simulink model "VXRv1 (1)"  (R2020b)
settings: Solver=VariableStepAuto  StartTime=0.0  StopTime=0.5  RelTol=1e-3
libraries: fl_lib x62, ee_lib x36, nesl_utility x19, powerlib_meascontrol x6
settings Model: Creator=Admin  LastModifiedBy=olivermizzaro

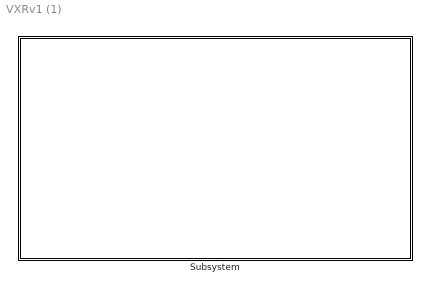
== system VXRv1 (1) ==
  Subsystem : Subsystem

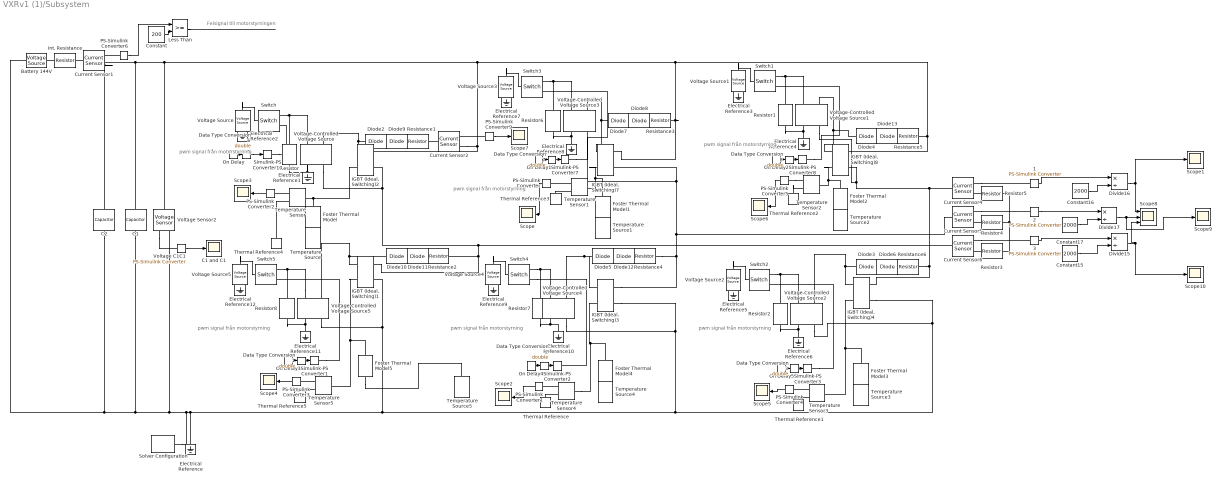
== system VXRv1 (1)/Subsystem ==
  note: pwm signal från motorstyrning
  note: Felsignal till motorstyrningen
  note: pwm signal från motorstyrning
  note: pwm signal från motorstyrning
  note: pwm signal från motorstyrning
  note: pwm signal från motorstyrning
  note: pwm signal från motorstyrning
   Resistance{1..6} (6 alike) : fl_lib/Electrical/Electrical Elements/Resistor  R=30 Ohm  i_specify=off  i_priority=None  i=0 A  i_nominal_specify=off  i_nominal_unit=A  i_nominal_value=1  v_specify=off  v_priority=None  v=0 V  v_nominal_specify=off  v_nominal_unit=V  v_nominal_value=1
  1 : nesl_utility/PS-Simulink Converter  PhysicalDomain=network_engine_domain  SubClassName=ps_output  LeftPortType=input  RightPortType=output  PseudoPeriodic=off  Frequencies=[]  Unit=inherit  AffineConversion=off
  2 : nesl_utility/PS-Simulink Converter  PhysicalDomain=network_engine_domain  SubClassName=ps_output  LeftPortType=input  RightPortType=output  PseudoPeriodic=off  Frequencies=[]  Unit=inherit  AffineConversion=off
  3 : nesl_utility/PS-Simulink Converter  PhysicalDomain=network_engine_domain  SubClassName=ps_output  LeftPortType=input  RightPortType=output  PseudoPeriodic=off  Frequencies=[]  Unit=inherit  AffineConversion=off
  Battery 144V : ee_lib/Sources/Voltage Source  dc_voltage=144 V  ac_voltage=0 V  ac_shift=0 rad  ac_frequency=60 Hz  noise_mode=0  PSD=0 V^2/Hz  repeatability=1  auto_seed=785646024  user_seed=0  sample_time=1e-3 s  i_specify=off  i_priority=None  i=0 A  i_nominal_specify=off  i_nominal_unit=A  i_nominal_value=1  v_specify=off  v_priority=None  v=0 V  v_nominal_specify=off  v_nominal_unit=V  v_nominal_value=1
  C1 : ee_lib/Passive/Capacitor  cap_option=0  c=10000e-6 F  Cvec=[1e-05, 1e-06] F  Vvec=[0, 10] V  CV_table_symmetry=1  f_vec=[1, 10] kHz  DFext_vec=[.8, 1.2]  C_tol=5  enable_C_tol=0  tol_distribution=1  nSigma=4  r=1 Ohm  g=0 1/Ohm  averaging_period=0 s  enable_operating_limits=0  operating_limit_action=2  max_working_voltage_range=[-25, 25] V  power_rating=1 W  enable_faults=0  fault_action=1  Cscale_faulted=100  R_faulted=1e-3 Ohm  G_faulted=0 1/Ohm  tau_fault=1e-3 s  enable_temporal_fault=0  t_fault=1 s  enable_behavioral_fault=0  max_permissible_voltage_range=[-100, 100] V  t_fail_on_voltage=1 s  i_specify=off  i_priority=None  i=0 A  i_nominal_specify=off  i_nominal_unit=A  i_nominal_value=1  v_specify=off  v_priority=None  v=0 V  v_nominal_specify=off  v_nominal_unit=V  v_nominal_value=1  vc_specify=on  vc_priority=High  vc=144 V  vc_nominal_specify=off  vc_nominal_unit=V  vc_nominal_value=1
  C1 and C1 : Scope
  C2 : ee_lib/Passive/Capacitor  cap_option=0  c=127e-9 F  Cvec=[1e-05, 1e-06] F  Vvec=[0, 10] V  CV_table_symmetry=1  f_vec=[1, 10] kHz  DFext_vec=[.8, 1.2]  C_tol=5  enable_C_tol=0  tol_distribution=1  nSigma=4  r=1 Ohm  g=0 1/Ohm  averaging_period=0 s  enable_operating_limits=0  operating_limit_action=2  max_working_voltage_range=[-25, 25] V  power_rating=1 W  enable_faults=0  fault_action=1  Cscale_faulted=100  R_faulted=1e-3 Ohm  G_faulted=0 1/Ohm  tau_fault=1e-3 s  enable_temporal_fault=0  t_fault=1 s  enable_behavioral_fault=0  max_permissible_voltage_range=[-100, 100] V  t_fail_on_voltage=1 s  i_specify=off  i_priority=None  i=0 A  i_nominal_specify=off  i_nominal_unit=A  i_nominal_value=1  v_specify=off  v_priority=None  v=0 V  v_nominal_specify=off  v_nominal_unit=V  v_nominal_value=1  vc_specify=off  vc_priority=High  vc=0 V  vc_nominal_specify=off  vc_nominal_unit=V  vc_nominal_value=1
  Constant : Constant  Value=200
  Constant15 : Constant  Value=2000
  Constant16 : Constant  Value=2000
  Constant17 : Constant  Value=2000
  Current Sensor{1..2,4..6} (5 alike) : fl_lib/Electrical/Electrical Sensors/Current Sensor
  Data Type Conversion{1..3,6..8} (6 alike) : DataTypeConversion  OutDataTypeStr=double
  Diode{2..5,7,10} (6 alike) : ee_lib/Semiconductors & Converters/Diode  ModelType=ee.enum.diode.modelType.pwl  IfMat=[.07, .12, .19, 1.75, 4.24, 7.32, 11.2; .16, .3, .72, 2.14, 4.02, 6.35, 9.12] A  TjVec=[25, 125] degC  VfVec=[.5, .7, .9, 1.3, 1.7, 2.1, 2.5] V  Vf=3 V  Ron=5 Ohm  Goff=1e-8 S  prmExp=ee.enum.diode.expParam.useTwo  I12=[.0137, .545] A  V12=[.6, .7] V  IS=1e-12 A  ec=1  I1=0.0137 A  V1=0.6 V  RS=0 Ohm  Tmeas=25 degC  N_series=1  N_parallel=1  Rz=1.5 Ohm  BV=150 V  C_param=ee.enum.diode.capParam.fixed  CJ=5 pF  CJ0=5 pF  VJ=1 V  Mgrad=0.5  Vvec=[.1, 10, 100] V  Cvec=[3.5, 1, .4] pF  FC=0.5  Q_param=ee.enum.diode.recoveryParam.off  iRM=-7.15 A  iF=4 A  didt=-750 A/us  trr_factor=3  trr=115 ns  Qrr=1500 s*uA  TT=50 ns  tau=100 ns  T_param=ee.enum.diode.temperatureParam.off  IS_T2=1.25e-7 A  I1_T2=0.245 A  V1_T2=0.5 V  Tmeas2=125 degC  EG_param=ee.enum.diode.egapParam.material_si  EG=1.11 eV  XTI_param=ee.enum.diode.xtiParam.pn  XTI=3  dBVdT=0 V/K  Tdevice=25 degC  i_specify=off  i_priority=None  i=0 A  i_nominal_specify=off  i_nominal_unit=A  i_nominal_value=1  v_specify=off  v_priority=None  v=0 V  v_nominal_specify=off  v_nominal_unit=V  v_nominal_value=1  i_capacitor_specify=off  i_capacitor_priority=None  i_capacitor=0 A  i_capacitor_nominal_specify=off  i_capacitor_nominal_unit=A  i_capacitor_nominal_value=1  v_capacitor_specify=off  v_capacitor_priority=None  v_capacitor=0 V  v_capacitor_nominal_specify=off  v_capacitor_nominal_unit=V  v_capacitor_nominal_value=1  power_dissipated_specify=off  power_dissipated_priority=None  power_dissipated=0 W  power_dissipated_nominal_specify=off  power_dissipated_nominal_unit=W  power_dissipated_nominal_value=1  thermal_network_parameterization=ee.enum.thermalNetworkTopology.cauer  Rth=[0, 10] K/W  Rth_Foster=[4, 6] K/W  thermal_mass_parameterization=ee.enum.thermalNetwork.timeconstant  thermal_mass=[0, 1] J/K  thermal_mass_Foster=[1.5, 3] J/K  thermal_time_constant=[0, 10] s  thermal_time_constant_Foster=[6, 18] s  thermal_mass_initial_temperatures=[25, 25] degC
  Diode{6,8..9,11..13} (6 alike) : ee_lib/Semiconductors & Converters/Diode  ModelType=ee.enum.diode.modelType.pwl  IfMat=[.07, .12, .19, 1.75, 4.24, 7.32, 11.2; .16, .3, .72, 2.14, 4.02, 6.35, 9.12] A  TjVec=[25, 125] degC  VfVec=[.5, .7, .9, 1.3, 1.7, 2.1, 2.5] V  Vf=0.6 V  Ron=0.3 Ohm  Goff=1e-8 S  prmExp=ee.enum.diode.expParam.useTwo  I12=[.0137, .545] A  V12=[.6, .7] V  IS=1e-12 A  ec=1  I1=0.0137 A  V1=0.6 V  RS=0 Ohm  Tmeas=25 degC  N_series=1  N_parallel=1  Rz=0.3 Ohm  BV=inf V  C_param=ee.enum.diode.capParam.fixed  CJ=5 pF  CJ0=5 pF  VJ=1 V  Mgrad=0.5  Vvec=[.1, 10, 100] V  Cvec=[3.5, 1, .4] pF  FC=0.5  Q_param=ee.enum.diode.recoveryParam.off  iRM=-7.15 A  iF=4 A  didt=-750 A/us  trr_factor=3  trr=115 ns  Qrr=1500 s*uA  TT=50 ns  tau=100 ns  T_param=ee.enum.diode.temperatureParam.off  IS_T2=1.25e-7 A  I1_T2=0.245 A  V1_T2=0.5 V  Tmeas2=125 degC  EG_param=ee.enum.diode.egapParam.material_si  EG=1.11 eV  XTI_param=ee.enum.diode.xtiParam.pn  XTI=3  dBVdT=0 V/K  Tdevice=25 degC  i_specify=off  i_priority=None  i=0 A  i_nominal_specify=off  i_nominal_unit=A  i_nominal_value=1  v_specify=off  v_priority=None  v=0 V  v_nominal_specify=off  v_nominal_unit=V  v_nominal_value=1  i_capacitor_specify=off  i_capacitor_priority=None  i_capacitor=0 A  i_capacitor_nominal_specify=off  i_capacitor_nominal_unit=A  i_capacitor_nominal_value=1  v_capacitor_specify=off  v_capacitor_priority=None  v_capacitor=0 V  v_capacitor_nominal_specify=off  v_capacitor_nominal_unit=V  v_capacitor_nominal_value=1  power_dissipated_specify=off  power_dissipated_priority=None  power_dissipated=0 W  power_dissipated_nominal_specify=off  power_dissipated_nominal_unit=W  power_dissipated_nominal_value=1  thermal_network_parameterization=ee.enum.thermalNetworkTopology.cauer  Rth=[0, 10] K/W  Rth_Foster=[4, 6] K/W  thermal_mass_parameterization=ee.enum.thermalNetwork.timeconstant  thermal_mass=[0, 1] J/K  thermal_mass_Foster=[1.5, 3] J/K  thermal_time_constant=[0, 10] s  thermal_time_constant_Foster=[6, 18] s  thermal_mass_initial_temperatures=[25, 25] degC
  Divide15 : Product  Inputs=*/
  Divide16 : Product  Inputs=*/
  Divide17 : Product  Inputs=*/
  Electrical Reference{,1..12} (13 alike) : fl_lib/Electrical/Electrical Elements/Electrical Reference
  Foster Thermal Model{,1..5} (6 alike) : ee_lib/Passive/Thermal/Foster Thermal Model  resistance_data=[ 0.0016 0.0043 0.0013 0.0014 ] K/W  tau_data=[ 0.0068 0.064 0.32 2 ] s
      settings: SourceProductBaseCode=PS  InternalSimscapePortConfiguration="{\"Bottom\":[],\"Left\":[{\"id\":\"A\",\"label\":\"A\",\"type\":\"foundation.thermal.thermal\"}],\"Right\":[{\"id\":\"B\",\"label\":\"B\",\"type\":\"foundation.thermal.thermal\"}],\"Top\":[]}"
  IGBT (Ideal, Switching){1,3..4,8} (4 alike) : ee_lib/Semiconductors & Converters/IGBT (Ideal, Switching)  Vf=1.5 V  Ron=0.001 Ohm  Goff=1e-5 1/Ohm  Vth=0.1 V  diode_param=ee.enum.converters.protectiondiode.none  diode_Vf=0.8 V  diode_Ron=0.001 Ohm  diode_Goff=1e-5 1/Ohm  diode_C=50e-9 F  diode_iRM=-235 A  diode_iF=300 A  diode_idot=-50 A/us  diode_trr_param=ee.enum.converters.diodetrr.trr_factor  diode_trr_factor=3  diode_trr=15 us  diode_Qrr=1500 s*uA  thermal_loss_option=ee.enum.converters.thermalLossOption.constantvalues  Von_data=[0, .1, .6, .8, 1, 1.3, 1.6, 2, 2.4; 0, .1, .7, 1, 1.2, 1.5, 1.9, 2.4, 2.8] V  Eon_data=[0, .0024, .024, .12, .2, .48, 1.04, 2.16, 3.24; 0, .003, .03, .15, .25, .6, 1.3, 2.7, 4.05] * 1e-3 J  Eoff_data=[0, .0007, .0066, .033, .066, .17, .33, .83, 1.5; 0, .001, .01, .05, .1, .25, .5, 1.2, 2.2] * 1e-3 J  Tj=[298.15, 398.15] K  Iout_data=[0, .1, 1, 5, 10, 20, 40, 70, 100] A  Eon_scalar=2.9e-3 J  Eoff_scalar=7.9e-3 J  Voff=300 V  Iout_scalar=600 A  diodeModelType=ee.enum.converters.diodeModelType.pwl  diode_IfMat=[.07, .12, .19, 1.75, 4.24, 7.32, 11.2; .16, .3, .72, 2.14, 4.02, 6.35, 9.12] A  diode_TjVec=[25, 125] degC  diode_VfVec=[.5, .7, .9, 1.3, 1.7, 2.1, 2.5] V  thermal_network_parameterization=ee.enum.thermalNetworkTopology.cauer  Rth=[.42, .06] K/W  Rth_Foster=[.08, .14, .22, .16] K/W  thermal_mass_parameterization=ee.enum.thermalNetwork.timeconstant  thermal_mass=[.01, .5] J/K  thermal_mass_Foster=[.001, .005, .05, .5] J/K  thermal_time_constant=[.001, .2] s  thermal_time_constant_Foster=[7e-05, .0007, .01, .08] s  thermal_mass_initial_temperatures=[25, 25] degC  junction_thermal_mass=0.01 J/K  Tau=1e-4 s  vT_specify=off  vT_priority=None  vT=0 V  vT_nominal_specify=off  vT_nominal_unit=V  vT_nominal_value=1  Qj_specify=off  Qj_priority=None  Qj=0 W  Qj_nominal_specify=off  Qj_nominal_unit=W  Qj_nominal_value=1  junction_temperature_specify=off  junction_temperature_priority=None  junction_temperature=25 degC  junction_temperature_nominal_specify=off  junction_temperature_nominal_unit=degC  junction_temperature_nominal_value=1
      settings: InternalSimscapePortConfiguration="{\"Bottom\":[],\"Left\":[{\"id\":\"G\",\"label\":\"\",\"type\":\"foundation.electrical.electrical\"},{\"id\":\"H\",\"label\":\"\",\"type\":\"foundation.thermal.thermal\"}],\"Right\":[{\"id\":\"C\",\"label\":\"\",\"type\":\"foundation.electrical.electrical\"},{\"id\":\"E\",\"label\":\"\",\"type\":\"foundation.electrical.electrical\"}],\"Top\":[]}"
  "IGBT (Ideal, Switching)2" : ee_lib/Semiconductors & Converters/IGBT (Ideal, Switching)  Vf=1.5 V  Ron=0.001 Ohm  Goff=1e-5 1/Ohm  Vth=7 V  diode_param=ee.enum.converters.protectiondiode.none  diode_Vf=0.8 V  diode_Ron=0.001 Ohm  diode_Goff=1e-5 1/Ohm  diode_C=50e-9 F  diode_iRM=-235 A  diode_iF=300 A  diode_idot=-50 A/us  diode_trr_param=ee.enum.converters.diodetrr.trr_factor  diode_trr_factor=3  diode_trr=15 us  diode_Qrr=1500 s*uA  thermal_loss_option=ee.enum.converters.thermalLossOption.constantvalues  Von_data=[0, .1, .6, .8, 1, 1.3, 1.6, 2, 2.4; 0, .1, .7, 1, 1.2, 1.5, 1.9, 2.4, 2.8] V  Eon_data=[0, .0024, .024, .12, .2, .48, 1.04, 2.16, 3.24; 0, .003, .03, .15, .25, .6, 1.3, 2.7, 4.05] * 1e-3 J  Eoff_data=[0, .0007, .0066, .033, .066, .17, .33, .83, 1.5; 0, .001, .01, .05, .1, .25, .5, 1.2, 2.2] * 1e-3 J  Tj=[298.15, 398.15] K  Iout_data=[0, .1, 1, 5, 10, 20, 40, 70, 100] A  Eon_scalar=2.9e-3 J  Eoff_scalar=7.9e-3 J  Voff=300 V  Iout_scalar=600 A  diodeModelType=ee.enum.converters.diodeModelType.pwl  diode_IfMat=[.07, .12, .19, 1.75, 4.24, 7.32, 11.2; .16, .3, .72, 2.14, 4.02, 6.35, 9.12] A  diode_TjVec=[25, 125] degC  diode_VfVec=[.5, .7, .9, 1.3, 1.7, 2.1, 2.5] V  thermal_network_parameterization=ee.enum.thermalNetworkTopology.cauer  Rth=[.42, .06] K/W  Rth_Foster=[.08, .14, .22, .16] K/W  thermal_mass_parameterization=ee.enum.thermalNetwork.timeconstant  thermal_mass=[.01, .5] J/K  thermal_mass_Foster=[.001, .005, .05, .5] J/K  thermal_time_constant=[.001, .2] s  thermal_time_constant_Foster=[7e-05, .0007, .01, .08] s  thermal_mass_initial_temperatures=[25, 25] degC  junction_thermal_mass=0.01 J/K  Tau=1e-4 s  vT_specify=off  vT_priority=None  vT=0 V  vT_nominal_specify=off  vT_nominal_unit=V  vT_nominal_value=1  Qj_specify=off  Qj_priority=None  Qj=0 W  Qj_nominal_specify=off  Qj_nominal_unit=W  Qj_nominal_value=1  junction_temperature_specify=off  junction_temperature_priority=None  junction_temperature=25 degC  junction_temperature_nominal_specify=off  junction_temperature_nominal_unit=degC  junction_temperature_nominal_value=1
      settings: InternalSimscapePortConfiguration="{\"Bottom\":[],\"Left\":[{\"id\":\"G\",\"label\":\"\",\"type\":\"foundation.electrical.electrical\"},{\"id\":\"H\",\"label\":\"\",\"type\":\"foundation.thermal.thermal\"}],\"Right\":[{\"id\":\"C\",\"label\":\"\",\"type\":\"foundation.electrical.electrical\"},{\"id\":\"E\",\"label\":\"\",\"type\":\"foundation.electrical.electrical\"}],\"Top\":[]}"
  "IGBT (Ideal, Switching)7" : ee_lib/Semiconductors & Converters/IGBT (Ideal, Switching)  Vf=1.5 V  Ron=0.001 Ohm  Goff=1e-5 1/Ohm  Vth=0.1 V  diode_param=ee.enum.converters.protectiondiode.none  diode_Vf=0.8 V  diode_Ron=0.001 Ohm  diode_Goff=1e-5 1/Ohm  diode_C=50e-9 F  diode_iRM=-235 A  diode_iF=300 A  diode_idot=-50 A/us  diode_trr_param=ee.enum.converters.diodetrr.trr_factor  diode_trr_factor=3  diode_trr=15 us  diode_Qrr=1500 s*uA  thermal_loss_option=ee.enum.converters.thermalLossOption.constantvalues  Von_data=[0, .1, .6, .8, 1, 1.3, 1.6, 2, 2.4; 0, .1, .7, 1, 1.2, 1.5, 1.9, 2.4, 2.8] V  Eon_data=[0, .0024, .024, .12, .2, .48, 1.04, 2.16, 3.24; 0, .003, .03, .15, .25, .6, 1.3, 2.7, 4.05] * 1e-3 J  Eoff_data=[0, .0007, .0066, .033, .066, .17, .33, .83, 1.5; 0, .001, .01, .05, .1, .25, .5, 1.2, 2.2] * 1e-3 J  Tj=[298.15, 398.15] K  Iout_data=[0, .1, 1, 5, 10, 20, 40, 70, 100] A  Eon_scalar=2.9e-3 J  Eoff_scalar=7.9e-3 J  Voff=300 V  Iout_scalar=600 A  diodeModelType=ee.enum.converters.diodeModelType.pwl  diode_IfMat=[.07, .12, .19, 1.75, 4.24, 7.32, 11.2; .16, .3, .72, 2.14, 4.02, 6.35, 9.12] A  diode_TjVec=[25, 125] degC  diode_VfVec=[.5, .7, .9, 1.3, 1.7, 2.1, 2.5] V  thermal_network_parameterization=ee.enum.thermalNetworkTopology.cauer  Rth=[.42, .06] K/W  Rth_Foster=[.08, .14, .22, .16] K/W  thermal_mass_parameterization=ee.enum.thermalNetwork.timeconstant  thermal_mass=[.01, .5] J/K  thermal_mass_Foster=[.001, .005, .05, .5] J/K  thermal_time_constant=[.001, .2] s  thermal_time_constant_Foster=[7e-05, .0007, .01, .08] s  thermal_mass_initial_temperatures=[25, 25] degC  junction_thermal_mass=0.01 J/K  Tau=1e-4 s  vT_specify=off  vT_priority=None  vT=0 V  vT_nominal_specify=off  vT_nominal_unit=V  vT_nominal_value=1  Qj_specify=off  Qj_priority=None  Qj=0 W  Qj_nominal_specify=off  Qj_nominal_unit=W  Qj_nominal_value=1  junction_temperature_specify=off  junction_temperature_priority=High  junction_temperature=25 degC  junction_temperature_nominal_specify=off  junction_temperature_nominal_unit=degC  junction_temperature_nominal_value=1
      settings: InternalSimscapePortConfiguration="{\"Bottom\":[],\"Left\":[{\"id\":\"G\",\"label\":\"\",\"type\":\"foundation.electrical.electrical\"},{\"id\":\"H\",\"label\":\"\",\"type\":\"foundation.thermal.thermal\"}],\"Right\":[{\"id\":\"C\",\"label\":\"\",\"type\":\"foundation.electrical.electrical\"},{\"id\":\"E\",\"label\":\"\",\"type\":\"foundation.electrical.electrical\"}],\"Top\":[]}"
  Int. Resistance : fl_lib/Electrical/Electrical Elements/Resistor  R=0.01 Ohm  i_specify=off  i_priority=None  i=0 A  i_nominal_specify=off  i_nominal_unit=A  i_nominal_value=1  v_specify=off  v_priority=None  v=0 V  v_nominal_specify=off  v_nominal_unit=V  v_nominal_value=1
  Less Than : RelationalOperator  OutDataTypeStr=boolean  RndMeth=Simplest
  On Delay{,1..5} (6 alike) : powerlib_meascontrol/Logic/On Delay  DelayType=On delay  delay=6e-6  ic=0  Ts=0
  PS-Simulink Converter{,1..6,9} (8 alike) : nesl_utility/PS-Simulink Converter  PhysicalDomain=network_engine_domain  SubClassName=ps_output  LeftPortType=input  RightPortType=output  PseudoPeriodic=off  Frequencies=[]  Unit=inherit  AffineConversion=off
  Resistor{,1..2,6..8} (6 alike) : fl_lib/Electrical/Electrical Elements/Resistor  R=1 Ohm  i_specify=off  i_priority=None  i=0 A  i_nominal_specify=off  i_nominal_unit=A  i_nominal_value=1  v_specify=off  v_priority=None  v=0 V  v_nominal_specify=off  v_nominal_unit=V  v_nominal_value=1
  Resistor3 : ee_lib/Passive/Resistor  R=0.5 Ohm  R_tol=5  enable_R_tol=0  tol_distribution=1  nSigma=4  enable_operating_limits=0  operating_limit_action=2  max_working_voltage=100 V  power_rating=1 W  enable_faults=0  fault_action=1  R_faulted=inf Ohm  enable_temporal_fault=0  t_fault=1 s  enable_behavioral_fault=0  max_permissible_current=1 A  t_fail_on_current=1 s  noise_mode=0  sample_time=1e-3 s  repeatability=1  auto_seed=2915145293  user_seed=0  Tdevice=25 degC  alpha=3.93e-3 1/K  Tmeas=25 degC  thermal_mass=100 J/K  power_derating_T1=70 degC  power_derating_T2=155 degC  operating_temperature_range_vec=[-50, 150] degC  temperature_specify=off  temperature_priority=High  temperature=298.15 K  temperature_nominal_specify=off  temperature_nominal_unit=K  temperature_nominal_value=1
  Resistor4 : ee_lib/Passive/Resistor  R=0.5 Ohm  R_tol=5  enable_R_tol=0  tol_distribution=1  nSigma=4  enable_operating_limits=0  operating_limit_action=2  max_working_voltage=100 V  power_rating=1 W  enable_faults=0  fault_action=1  R_faulted=inf Ohm  enable_temporal_fault=0  t_fault=1 s  enable_behavioral_fault=0  max_permissible_current=1 A  t_fail_on_current=1 s  noise_mode=0  sample_time=1e-3 s  repeatability=1  auto_seed=3254469079  user_seed=0  Tdevice=25 degC  alpha=3.93e-3 1/K  Tmeas=25 degC  thermal_mass=100 J/K  power_derating_T1=70 degC  power_derating_T2=155 degC  operating_temperature_range_vec=[-50, 150] degC  temperature_specify=off  temperature_priority=High  temperature=298.15 K  temperature_nominal_specify=off  temperature_nominal_unit=K  temperature_nominal_value=1
  Resistor5 : ee_lib/Passive/Resistor  R=0.5 Ohm  R_tol=5  enable_R_tol=0  tol_distribution=1  nSigma=4  enable_operating_limits=0  operating_limit_action=2  max_working_voltage=100 V  power_rating=1 W  enable_faults=0  fault_action=1  R_faulted=inf Ohm  enable_temporal_fault=0  t_fault=1 s  enable_behavioral_fault=0  max_permissible_current=1 A  t_fail_on_current=1 s  noise_mode=0  sample_time=1e-3 s  repeatability=1  auto_seed=3191729647  user_seed=0  Tdevice=25 degC  alpha=3.93e-3 1/K  Tmeas=25 degC  thermal_mass=100 J/K  power_derating_T1=70 degC  power_derating_T2=155 degC  operating_temperature_range_vec=[-50, 150] degC  temperature_specify=off  temperature_priority=High  temperature=298.15 K  temperature_nominal_specify=off  temperature_nominal_unit=K  temperature_nominal_value=1
  Scope{,1..7,9..10} (10 alike) : Scope
  Scope8 : Scope  NumInputPorts=3
  Simulink-PS Converter{1..3,7..8,10} (6 alike) : nesl_utility/Simulink-PS Converter  PhysicalDomain=network_engine_domain  SubClassName=ps_input  LeftPortType=input  RightPortType=output  PseudoPeriodic=off  Frequencies=[]  NoiseDistribution=none  NoiseParameters=[]  Unit=1  AffineConversion=off  FilteringAndDerivatives=provide  SimscapeFilterOrder=1  InputFilterTimeConstant=0.001  UdotUserProvided=0
  Solver Configuration : nesl_utility/Solver Configuration  PhysicalDomain=network_engine_domain  SubClassName=solver  LeftPortType=input  RightPortType=generic  Tones=[]  Harmonics=[]  SimulateNoise=off  Profile=off  UseLocalSampling=off  EnableSwitchedLinearOptims=on  FrequencyDomain=off  UseCCode=off  RelTol=0.001  AbsTol=1e-06  MinStep=1e-09  ToWorkspace=off  RevertToSquareIcSolve=off  NumHomotopyIterations=100  PhasorMode=off  PhasorModeNumHarmonics=1  DoDC=off  ResidualTolerance=1e-09  UseLocalSolver=off  LocalSolverChoice=NE_BACKWARD_EULER_ADVANCER  LocalSolverSampleTime=0.001  DoFixedCost=off  MaxNonlinIter=3  MaxModeIter=2  ComputeImpulses=off  ImpulseIterations=2  LinearAlgebra=auto  EquationFormulation=NE_TIME_EF  DelaysMemoryBudget=1024  AutomaticFiltering=on  FilteringTimeConstant=0.001  PartitionStorageMethod=AS_NEEDED  PartitionMemoryBudget=1024  PartitionMethod=ROBUST
  Switch{,1..5} (6 alike) : fl_lib/Electrical/Electrical Elements/Switch  R_closed=0.01 Ohm  G_open=1e-8 1/Ohm  Threshold=0.5  i_specify=off  i_priority=None  i=0 A  i_nominal_specify=off  i_nominal_unit=A  i_nominal_value=1  v_specify=off  v_priority=None  v=0 V  v_nominal_specify=off  v_nominal_unit=V  v_nominal_value=1
  Temperature Sensor{,1..5} (6 alike) : fl_lib/Thermal/Thermal Sensors/Temperature Sensor
  Temperature Source{,1..5} (6 alike) : fl_lib/Thermal/Thermal Sources/Temperature Source  temperature=298.15 K
  Thermal Reference{,1..5} (6 alike) : fl_lib/Thermal/Thermal Elements/Thermal Reference
  Voltage C1C1 : nesl_utility/PS-Simulink Converter  PhysicalDomain=network_engine_domain  SubClassName=ps_output  LeftPortType=input  RightPortType=output  PseudoPeriodic=off  Frequencies=[]  Unit=inherit  AffineConversion=off
  Voltage Sensor2 : fl_lib/Electrical/Electrical Sensors/Voltage Sensor
  Voltage Source : ee_lib/Sources/Voltage Source  dc_voltage=1 V  ac_voltage=0 V  ac_shift=0 rad  ac_frequency=60 Hz  noise_mode=0  PSD=0 V^2/Hz  repeatability=1  auto_seed=3961385766  user_seed=0  sample_time=1e-3 s  i_specify=off  i_priority=None  i=0 A  i_nominal_specify=off  i_nominal_unit=A  i_nominal_value=1  v_specify=off  v_priority=None  v=0 V  v_nominal_specify=off  v_nominal_unit=V  v_nominal_value=1
  Voltage Source1 : ee_lib/Sources/Voltage Source  dc_voltage=1 V  ac_voltage=0 V  ac_shift=0 rad  ac_frequency=60 Hz  noise_mode=0  PSD=0 V^2/Hz  repeatability=1  auto_seed=3439496942  user_seed=0  sample_time=1e-3 s  i_specify=off  i_priority=None  i=0 A  i_nominal_specify=off  i_nominal_unit=A  i_nominal_value=1  v_specify=off  v_priority=None  v=0 V  v_nominal_specify=off  v_nominal_unit=V  v_nominal_value=1
  Voltage Source2 : ee_lib/Sources/Voltage Source  dc_voltage=1 V  ac_voltage=0 V  ac_shift=0 rad  ac_frequency=60 Hz  noise_mode=0  PSD=0 V^2/Hz  repeatability=1  auto_seed=4212949037  user_seed=0  sample_time=1e-3 s  i_specify=off  i_priority=None  i=0 A  i_nominal_specify=off  i_nominal_unit=A  i_nominal_value=1  v_specify=off  v_priority=None  v=0 V  v_nominal_specify=off  v_nominal_unit=V  v_nominal_value=1
  Voltage Source3 : ee_lib/Sources/Voltage Source  dc_voltage=1 V  ac_voltage=0 V  ac_shift=0 rad  ac_frequency=60 Hz  noise_mode=0  PSD=0 V^2/Hz  repeatability=1  auto_seed=1231025197  user_seed=0  sample_time=1e-3 s  i_specify=off  i_priority=None  i=0 A  i_nominal_specify=off  i_nominal_unit=A  i_nominal_value=1  v_specify=off  v_priority=None  v=0 V  v_nominal_specify=off  v_nominal_unit=V  v_nominal_value=1
  Voltage Source4 : ee_lib/Sources/Voltage Source  dc_voltage=1 V  ac_voltage=0 V  ac_shift=0 rad  ac_frequency=60 Hz  noise_mode=0  PSD=0 V^2/Hz  repeatability=1  auto_seed=3848768948  user_seed=0  sample_time=1e-3 s  i_specify=off  i_priority=None  i=0 A  i_nominal_specify=off  i_nominal_unit=A  i_nominal_value=1  v_specify=off  v_priority=None  v=0 V  v_nominal_specify=off  v_nominal_unit=V  v_nominal_value=1
  Voltage Source5 : ee_lib/Sources/Voltage Source  dc_voltage=1 V  ac_voltage=0 V  ac_shift=0 rad  ac_frequency=60 Hz  noise_mode=0  PSD=0 V^2/Hz  repeatability=1  auto_seed=2566357106  user_seed=0  sample_time=1e-3 s  i_specify=off  i_priority=None  i=0 A  i_nominal_specify=off  i_nominal_unit=A  i_nominal_value=1  v_specify=off  v_priority=None  v=0 V  v_nominal_specify=off  v_nominal_unit=V  v_nominal_value=1
  Voltage-Controlled Voltage Source{,1..5} (6 alike) : fl_lib/Electrical/Electrical Sources/Voltage-Controlled Voltage Source  K=15  v1_specify=off  v1_priority=None  v1=0 V  v1_nominal_specify=off  v1_nominal_unit=V  v1_nominal_value=1  v2_specify=off  v2_priority=None  v2=0 V  v2_nominal_specify=off  v2_nominal_unit=V  v2_nominal_value=1
      settings: SourceProductBaseCode=SS  InternalSimscapePortConfiguration="{\"Bottom\":[],\"Left\":[{\"id\":\"p1\",\"label\":\"+\",\"type\":\"foundation.electrical.electrical\"},{\"id\":\"p2\",\"label\":\"+\",\"type\":\"foundation.electrical.electrical\"}],\"Right\":[{\"id\":\"n1\",\"label\":\"-\",\"type\":\"foundation.electrical.electrical\"},{\"id\":\"n2\",\"label\":\"-\",\"type\":\"foundation.electrical.electrical\"}],\"Top\":[]}"
  wires:
  ? -> On Delay/1
  Data Type Conversion6/1 -> Simulink-PS Converter10/1
  ? -> On Delay1/1
  Data Type Conversion7/1 -> Simulink-PS Converter7/1
  ? -> On Delay2/1
  Data Type Conversion8/1 -> Simulink-PS Converter8/1
  On Delay/1 -> Data Type Conversion6/1
  On Delay1/1 -> Data Type Conversion7/1
  On Delay2/1 -> Data Type Conversion8/1
  Voltage C1C1/1 -> C1 and C1/1
  ? -> On Delay3/1
  ? -> On Delay4/1
  On Delay3/1 -> Data Type Conversion1/1
  Data Type Conversion3/1 -> Simulink-PS Converter3/1
  Data Type Conversion1/1 -> Simulink-PS Converter1/1
  On Delay5/1 -> Data Type Conversion3/1
  Data Type Conversion2/1 -> Simulink-PS Converter2/1
  On Delay4/1 -> Data Type Conversion2/1
  ? -> On Delay5/1
  PS-Simulink Converter/1 -> Scope/1
  PS-Simulink Converter2/1 -> Scope3/1
  PS-Simulink Converter3/1 -> Scope4/1
  PS-Simulink Converter1/1 -> Scope2/1
  PS-Simulink Converter4/1 -> Scope5/1
  PS-Simulink Converter5/1 -> Scope6/1
  Constant/1 -> Less Than/2
  Divide17/1 -> Scope9/1, Scope8/2
  2/1 -> Divide17/1
  Constant15/1 -> Divide15/2
  3/1 -> Divide15/1
  Divide16/1 -> Scope8/1, Scope1/1
  Constant16/1 -> Divide16/2
  1/1 -> Divide16/1
  Divide15/1 -> Scope8/3, Scope10/1
  Constant17/1 -> Divide17/2
  PS-Simulink Converter9/1 -> Scope7/1
  PS-Simulink Converter6/1 -> Less Than/1
  Less Than/1 -> ?
  connections:
  Resistor4/LConn1 -- Current Sensor5/RConn2
  Resistor3/LConn1 -- Current Sensor6/RConn2
  Current Sensor4/RConn2 -- Resistor5/LConn1
  Voltage Sensor2/RConn1 -- Voltage C1C1/LConn1
  Battery 144V/LConn1 -- Int. Resistance/LConn1
  "IGBT (Ideal, Switching)8"/RConn2 -- Voltage-Controlled Voltage Source1/RConn2 -- Current Sensor4/LConn1 -- " Resistance6"/RConn1 -- "IGBT (Ideal, Switching)4"/RConn1
  "IGBT (Ideal, Switching)3"/RConn1 -- " Resistance4"/RConn1 -- Voltage-Controlled Voltage Source3/RConn2 -- "IGBT (Ideal, Switching)7"/RConn2 -- Current Sensor5/LConn1
  "IGBT (Ideal, Switching)1"/RConn1 -- " Resistance2"/RConn1 -- Voltage-Controlled Voltage Source/RConn2 -- "IGBT (Ideal, Switching)2"/RConn2 -- Current Sensor6/LConn1
  Temperature Sensor4/LConn1 -- Foster Thermal Model4/LConn1 -- "IGBT (Ideal, Switching)3"/LConn2
  Temperature Sensor4/RConn1 -- Thermal Reference/LConn1
  "IGBT (Ideal, Switching)4"/LConn2 -- Foster Thermal Model3/LConn1 -- Temperature Sensor3/LConn1
  Temperature Sensor3/RConn1 -- Thermal Reference1/LConn1
  "IGBT (Ideal, Switching)8"/LConn2 -- Foster Thermal Model2/LConn1 -- Temperature Sensor2/LConn1
  Thermal Reference2/LConn1 -- Temperature Sensor2/RConn1
  "IGBT (Ideal, Switching)7"/LConn2 -- Foster Thermal Model1/LConn1 -- Temperature Sensor1/LConn1
  Foster Thermal Model/LConn1 -- "IGBT (Ideal, Switching)2"/LConn2 -- Temperature Sensor/LConn1
  Temperature Sensor5/RConn1 -- Thermal Reference5/LConn1
  "IGBT (Ideal, Switching)1"/LConn2 -- Foster Thermal Model5/LConn1 -- Temperature Sensor5/LConn1
  Resistor5/RConn1 -- Resistor3/RConn1 -- Resistor4/RConn1
  Current Sensor5/RConn1 -- 2/LConn1
  Current Sensor6/RConn1 -- 3/LConn1
  Current Sensor4/RConn1 -- 1/LConn1
  Temperature Sensor1/RConn2 -- PS-Simulink Converter/LConn1
  Temperature Sensor1/RConn1 -- Thermal Reference3/LConn1
  Temperature Sensor/RConn2 -- PS-Simulink Converter2/LConn1
  Temperature Sensor5/RConn2 -- PS-Simulink Converter3/LConn1
  Temperature Sensor3/RConn2 -- PS-Simulink Converter4/LConn1
  PS-Simulink Converter5/LConn1 -- Temperature Sensor2/RConn2
  Temperature Sensor4/RConn2 -- PS-Simulink Converter1/LConn1
  C2/RConn1 -- Battery 144V/RConn1 -- C1/RConn1 -- Voltage Sensor2/RConn2 -- Solver Configuration/RConn1 -- Electrical Reference/LConn1 -- Voltage-Controlled Voltage Source2/RConn2 -- "IGBT (Ideal, Switching)4"/RConn2 -- Voltage-Controlled Voltage Source4/RConn2 -- "IGBT (Ideal, Switching)3"/RConn2 -- Voltage-Controlled Voltage Source5/RConn2 -- "IGBT (Ideal, Switching)1"/RConn2
  Foster Thermal Model/RConn1 -- Temperature Source/LConn1
  Temperature Sensor/RConn1 -- Thermal Reference4/LConn1
  Voltage-Controlled Voltage Source/LConn2 -- Diode2/LConn1 -- "IGBT (Ideal, Switching)2"/LConn1
  Electrical Reference1/LConn1 -- Resistor/RConn1 -- Voltage-Controlled Voltage Source/RConn1
  Electrical Reference2/LConn1 -- Voltage Source/RConn1
  Voltage Source/LConn1 -- Switch/LConn1
  Resistor/LConn1 -- Switch/RConn2 -- Voltage-Controlled Voltage Source/LConn1
  Simulink-PS Converter10/RConn1 -- Switch/RConn1
  Voltage-Controlled Voltage Source2/LConn1 -- Resistor2/LConn1 -- Switch2/RConn2
  Resistor2/RConn1 -- Electrical Reference6/LConn1 -- Voltage-Controlled Voltage Source2/RConn1
  Electrical Reference5/LConn1 -- Voltage Source2/RConn1
  Voltage Source2/LConn1 -- Switch2/LConn1
  Resistor6/LConn1 -- Voltage-Controlled Voltage Source3/LConn1 -- Switch3/RConn2
  Electrical Reference8/LConn1 -- Resistor6/RConn1 -- Voltage-Controlled Voltage Source3/RConn1
  Voltage Source3/LConn1 -- Switch3/LConn1
  Electrical Reference7/LConn1 -- Voltage Source3/RConn1
  Voltage Sensor2/LConn1 -- " Resistance3"/RConn1 -- "IGBT (Ideal, Switching)7"/RConn1 -- "IGBT (Ideal, Switching)8"/RConn1 -- " Resistance5"/RConn1 -- Current Sensor2/RConn2 -- "IGBT (Ideal, Switching)2"/RConn1 -- Current Sensor1/RConn2 -- C2/LConn1 -- C1/LConn1
  Simulink-PS Converter7/RConn1 -- Switch3/RConn1
  Voltage-Controlled Voltage Source3/LConn2 -- Diode7/LConn1 -- "IGBT (Ideal, Switching)7"/LConn1
  Resistor1/LConn1 -- Voltage-Controlled Voltage Source1/LConn1 -- Switch1/RConn2
  Electrical Reference4/LConn1 -- Resistor1/RConn1 -- Voltage-Controlled Voltage Source1/RConn1
  Voltage Source1/LConn1 -- Switch1/LConn1
  Electrical Reference3/LConn1 -- Voltage Source1/RConn1
  Simulink-PS Converter8/RConn1 -- Switch1/RConn1
  "IGBT (Ideal, Switching)8"/LConn1 -- Diode4/LConn1 -- Voltage-Controlled Voltage Source1/LConn2
  Resistor7/LConn1 -- Switch4/RConn2 -- Voltage-Controlled Voltage Source4/LConn1
  Electrical Reference10/LConn1 -- Resistor7/RConn1 -- Voltage-Controlled Voltage Source4/RConn1
  Voltage Source4/LConn1 -- Switch4/LConn1
  Electrical Reference9/LConn1 -- Voltage Source4/RConn1
  Voltage-Controlled Voltage Source5/LConn1 -- Resistor8/LConn1 -- Switch5/RConn2
  Resistor8/RConn1 -- Electrical Reference11/LConn1 -- Voltage-Controlled Voltage Source5/RConn1
  Electrical Reference12/LConn1 -- Voltage Source5/RConn1
  Voltage Source5/LConn1 -- Switch5/LConn1
  Simulink-PS Converter3/RConn1 -- Switch2/RConn1
  Voltage-Controlled Voltage Source2/LConn2 -- Diode3/LConn1 -- "IGBT (Ideal, Switching)4"/LConn1
  Voltage-Controlled Voltage Source4/LConn2 -- "IGBT (Ideal, Switching)3"/LConn1 -- Diode5/LConn1
  Switch4/RConn1 -- Simulink-PS Converter2/RConn1
  Simulink-PS Converter1/RConn1 -- Switch5/RConn1
  Voltage-Controlled Voltage Source5/LConn2 -- Diode10/LConn1 -- "IGBT (Ideal, Switching)1"/LConn1
  Foster Thermal Model1/RConn1 -- Temperature Source1/LConn1
  Foster Thermal Model2/RConn1 -- Temperature Source2/LConn1
  Foster Thermal Model3/RConn1 -- Temperature Source3/LConn1
  Foster Thermal Model4/RConn1 -- Temperature Source4/LConn1
  Foster Thermal Model5/RConn1 -- Temperature Source5/LConn1
  Diode8/RConn1 -- Diode7/RConn1
  Diode8/LConn1 -- " Resistance3"/LConn1
  Diode9/RConn1 -- Diode2/RConn1
  Diode9/LConn1 -- " Resistance1"/LConn1
  Diode11/RConn1 -- Diode10/RConn1
  Diode11/LConn1 -- " Resistance2"/LConn1
  Diode12/RConn1 -- Diode5/RConn1
  Diode12/LConn1 -- " Resistance4"/LConn1
  Diode13/RConn1 -- Diode4/RConn1
  Diode13/LConn1 -- " Resistance5"/LConn1
  Diode6/RConn1 -- Diode3/RConn1
  Diode6/LConn1 -- " Resistance6"/LConn1
  Current Sensor2/LConn1 -- " Resistance1"/RConn1
  PS-Simulink Converter9/LConn1 -- Current Sensor2/RConn1
  Current Sensor1/LConn1 -- Int. Resistance/RConn1
  PS-Simulink Converter6/LConn1 -- Current Sensor1/RConn1
